simulink model "MATE_SynchronousMachineV2"  (R2024b)
settings: Solver=FixedStepDiscrete  StartTime=0.0  StopTime=6  FixedStep=Ts  RelTol=1e-4  EnableMultiTasking=on
PostLoadFcn:
  | Ts=25e-6;offset=4;
InitFcn:
  | Ts=25e-6;offset=4;
undefined symbols (not defined in the file): DiscIntNeverNeededParam, MATE, Phase, Rsnu, Single
libraries: fl_lib x76, nesl_utility x63, ee_lib x16, artemis x9, simetran x5, powerlib_extras x3, simulink_extras x2, simulink x2
(part 4 of 5)

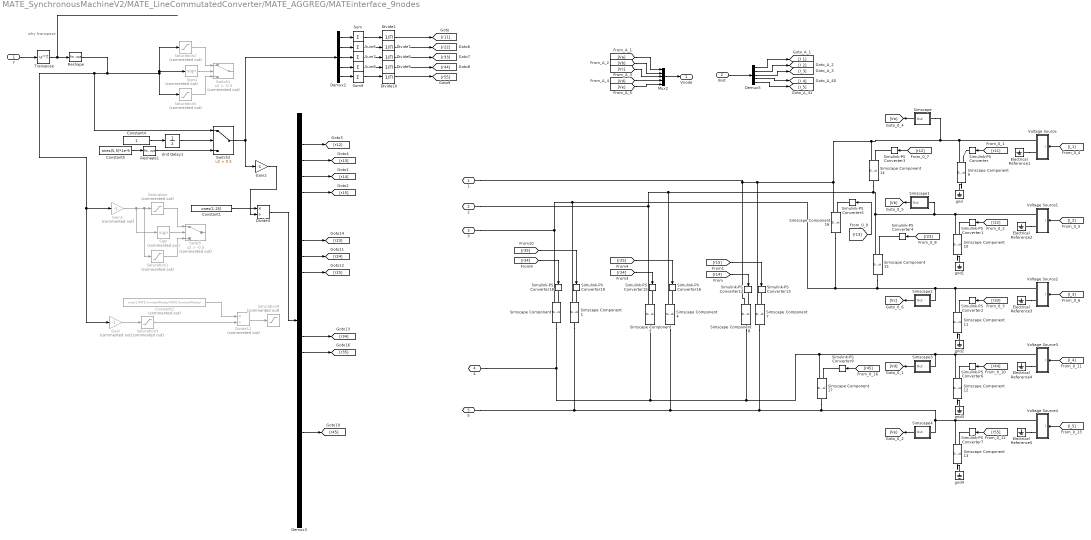
== system MATE_SynchronousMachineV2/MATE_LineCommutatedConverter/MATE_AGGREG/MATEinterface_9nodes ==
  note: why transpose
  Y : Inport
  Ihist : Inport  Port=2
  Constant1 : Constant  Value=ones(1,25)
  Constant2 : Constant  Commented=on  Value=ones(1,MATE.NumberOfNodes*MATE.NumberOfNodes)
  Constant4 : Constant
  Constant5 : Constant  Value=ones(5,5)*1e-9
  Demux2 : Demux  Outputs=[5 5 5 5 5]
      settings: DisplayOption=none
  Demux3 : Demux  Outputs=25
      settings: DisplayOption=none
  Demux5 : Demux  Outputs=[1 1 1 1 1]
      settings: DisplayOption=none
  Divide{1,7..10} (5 alike) : Product  Inputs=/
  Divide12 : Product  Commented=on  Inputs=*/  CollapseMode=Specified dimension
  Divide4 : Product  Inputs=*/  CollapseMode=Specified dimension
  Electrical Reference{1..5} (5 alike) : fl_lib/Electrical/Electrical Elements/Electrical Reference
  Gain : Gain  Commented=on  Gain=-1
  Gain1 : Gain  Commented=on  Gain=-1
  Gain2 : Gain  Gain=-1
  Mux2 : Mux  Inputs=[1 1 1 1 1]
  Reshape : Reshape
  Reshape1 : Reshape
  Saturation : Saturate  Commented=on  UpperLimit=1e12  LowerLimit=1e-12
  Saturation1 : Saturate  Commented=on  UpperLimit=-1e-12  LowerLimit=-1e12
  Saturation2 : Saturate  Commented=on  UpperLimit=1e12  LowerLimit=1e-12
  Saturation3 : Saturate  Commented=on  UpperLimit=1e15  LowerLimit=-1e15
  Saturation4 : Saturate  Commented=on  UpperLimit=1e15  LowerLimit=-1e15
  Saturation5 : Saturate  Commented=on  UpperLimit=-1e-12  LowerLimit=-1e12
  Sign : Signum  Commented=on
  Sign1 : Signum  Commented=on
  Simscape : Subsystem
      mask Display: disp('V')
  Simscape Component{,1,3..4,7..17} (15 alike) : SimscapeComponentBlock  SourceFile=variable_resistor_unlimited  ComponentPath=variable_resistor_unlimited  ComponentVariants="[\"variable_resistor_unlimited\"]"  ComponentVariantNames="[\"variable_resistor_unlimited\"]"  ClassName=variable_resistor_unlimited  SchemaVersion=1  R0=0 Ohm  Rmaxp=1e9 Ohm  Rmaxn=-1e9 Ohm  Rminp=1e-9 Ohm  Rminn=-1e-9 Ohm  i_specify=off  i_priority=None  i=0 A  i_nominal_specify=off  i_nominal_value=1  i_nominal_unit=A  v_specify=off  v_priority=None  v=0 V  v_nominal_specify=off  v_nominal_value=1  v_nominal_unit=V
      settings: CopyFcn=simscape.engine.sli.internal.componentblockcallback(gcbh,'COPY')  PreCopyFcn=simscape.engine.sli.internal.componentblockcallback(gcbh,'PRECOPY')  PreDeleteFcn=simscape.engine.sli.internal.componentblockcallback(gcbh,'PREDELETE')  InternalSimscapePortConfiguration="{\"Bottom\":[],\"Left\":[{\"id\":\"R\",\"label\":\"R\",\"type\":\"input\"},{\"id\":\"p\",\"label\":\"+\",\"type\":\"foundation.electrical.electrical\"}],\"Right\":[{\"id\":\"n\",\"label\":\"-\",\"type\":\"foundation.electrical.electrical\"}],\"Top\":[]}"
      mask Type: Variable Resistor
  Simscape1 : Subsystem
      mask Display: disp('V')
  Simscape2 : Subsystem
      mask Display: disp('V')
  Simscape3 : Subsystem
      mask Display: disp('V')
  Simscape4 : Subsystem
      mask Display: disp('V')
  Simulink-PS Converter{,1..7,9,12..13,15..16,18..19} (15 alike) : nesl_utility/Simulink-PS Converter  PhysicalDomain=network_engine_domain  SubClassName=ps_input  LeftPortType=input  RightPortType=output  PseudoPeriodic=off  Frequencies=[]  NoiseDistribution=none  NoiseParameters=[]  Unit=1  AffineConversion=off  FilteringAndDerivatives=provide  SimscapeFilterOrder=1  InputFilterTimeConstant=0.001  UdotUserProvided=0
  Sum{,6..9} (5 alike) : Sum  Inputs=+
  Switch : Switch  Commented=on  Criteria=u2 > Threshold  Threshold=-0.5  SaturateOnIntegerOverflow=off  InputSameDT=off
  Switch1 : Switch  Commented=on  Criteria=u2 > Threshold  Threshold=-0.5  SaturateOnIntegerOverflow=off  InputSameDT=off
  Switch2 : Switch  Criteria=u2 > Threshold  Threshold=0.5  SaturateOnIntegerOverflow=off  InputSameDT=off
  Transpose : Math  Operator=transpose
  Unit Delay1 : UnitDelay  SampleTime=Ts  HasFrameUpgradeWarning=on
  Voltage Source : Subsystem
  Voltage Source1 : Subsystem
  Voltage Source2 : Subsystem
  Voltage Source3 : Subsystem
  Voltage Source4 : Subsystem
  gnd{,1..4} (5 alike) : fl_lib/Electrical/Electrical Elements/Electrical Reference
  1 : PMIOPort  Side=Right
  2 : PMIOPort  Port=2  Side=Right
  3 : PMIOPort  Port=3  Side=Right
  4 : PMIOPort  Port=4  Side=Right
  5 : PMIOPort  Port=5  Side=Right
  Vnode : Outport  VectorParamsAs1DForOutWhenUnconnected=off
  wires:
  [I_2] -> Voltage Source1/1(I)
  Simscape2/1(Out) -> [Vc]
  [I_3] -> Voltage Source2/1(I)
  Simscape/1(Out) -> [Va]
  Simscape1/1(Out) -> [Vb]
  [I_1] -> Voltage Source/1(I)
  Y/1 -> Transpose/1
  Transpose/1 -> Reshape/1
  [r11] -> Simulink-PS Converter/1
  Sum/1 -> Divide1/1
  Divide1/1 -> [r11]
  [r22] -> Simulink-PS Converter1/1
  [r33] -> Simulink-PS Converter2/1
  [r12] -> Simulink-PS Converter3/1
  [r23] -> Simulink-PS Converter4/1
  [r13] -> Simulink-PS Converter5/1
  Demux2/1 -> Sum/1
  Divide7/1 -> [r22]
  Sum6/1 -> Divide7/1
  Demux2/2 -> Sum6/1
  Sum7/1 -> Divide8/1
  Divide8/1 -> [r33]
  Demux2/3 -> Sum7/1
  Demux2/4 -> Sum8/1
  Divide9/1 -> [r44]
  Sum8/1 -> Divide9/1
  Sum9/1 -> Divide10/1
  Divide10/1 -> [r55]
  Demux2/5 -> Sum9/1
  [r44] -> Simulink-PS Converter6/1
  [I_4] -> Voltage Source3/1(I)
  Simscape3/1(Out) -> [Vd]
  Simscape4/1(Out) -> [Ve]
  [I_5] -> Voltage Source4/1(I)
  [r55] -> Simulink-PS Converter7/1
  [r45] -> Simulink-PS Converter9/1
  [r14] -> Simulink-PS Converter12/1
  [r15] -> Simulink-PS Converter13/1
  [r25] -> Simulink-PS Converter16/1
  [r24] -> Simulink-PS Converter15/1
  Mux2/1 -> Vnode/1
  Ihist/1 -> Demux5/1
  Demux3/2 -> [r12]
  Demux3/3 -> [r13]
  Demux3/4 -> [r14]
  Demux3/5 -> [r15]
  Gain1/1 -> Sign/1, Saturation1/1, Saturation/1
  Constant1/1 -> Divide4/1
  [r35] -> Simulink-PS Converter19/1
  [r34] -> Simulink-PS Converter18/1
  Sign/1 -> Switch/2
  Saturation/1 -> Switch/1
  Saturation1/1 -> Switch/3
  Divide12/1 -> Saturation4/1
  Saturation3/1 -> Divide12/2
  Constant2/1 -> Divide12/1
  Gain/1 -> Saturation3/1
  Saturation5/1 -> Switch1/3
  Saturation2/1 -> Switch1/1
  Sign1/1 -> Switch1/2
  Reshape/1 -> Gain1/1, Gain/1, Switch2/1, Saturation2/1, Sign1/1, Saturation5/1
  Unit Delay1/1 -> Switch2/2
  Constant4/1 -> Unit Delay1/1
  Reshape1/1 -> Switch2/3
  Gain2/1 -> Divide4/2
  Demux5/4 -> [I_4]
  Demux5/3 -> [I_3]
  Demux5/5 -> [I_5]
  Demux5/2 -> [I_2]
  Demux5/1 -> [I_1]
  [Vd] -> Mux2/4
  [Ve] -> Mux2/5
  [Vc] -> Mux2/3
  [Vb] -> Mux2/2
  [Va] -> Mux2/1
  Demux3/8 -> [r23]
  Demux3/9 -> [r24]
  Demux3/10 -> [r25]
  Demux3/14 -> [r34]
  Demux3/15 -> [r35]
  Demux3/20 -> [r45]
  Constant5/1 -> Reshape1/1
  Switch2/1 -> Demux2/1, Gain2/1
  Divide4/1 -> Demux3/1
  connections:
  Simscape Component14/LConn2 -- Simscape Component9/LConn2 -- Voltage Source/RConn1 -- Simscape/LConn1 -- Simscape Component16/LConn2 -- Simscape Component7/LConn2 -- 1/RConn1 -- Simscape Component8/LConn2
  Simscape Component11/LConn2 -- Voltage Source2/RConn1 -- Simscape2/LConn1 -- Simscape Component15/RConn1 -- Simscape Component16/RConn1 -- Simscape Component1/LConn2 -- Simscape Component/LConn2 -- 3/RConn1
  Simscape Component10/LConn2 -- Voltage Source1/RConn1 -- Simscape1/LConn1 -- Simscape Component15/LConn2 -- Simscape Component14/RConn1 -- Simscape Component4/LConn2 -- Simscape Component3/LConn2 -- 2/RConn1
  Electrical Reference2/LConn1 -- Voltage Source1/RConn2
  Electrical Reference3/LConn1 -- Voltage Source2/RConn2
  Electrical Reference1/LConn1 -- Voltage Source/RConn2
  Simscape Component9/RConn1 -- gnd/LConn1
  Simscape Component9/LConn1 -- Simulink-PS Converter/RConn1
  Simscape Component10/RConn1 -- gnd1/LConn1
  Simscape Component10/LConn1 -- Simulink-PS Converter1/RConn1
  Simscape Component11/RConn1 -- gnd2/LConn1
  Simscape Component11/LConn1 -- Simulink-PS Converter2/RConn1
  Simscape Component14/LConn1 -- Simulink-PS Converter3/RConn1
  Simscape Component15/LConn1 -- Simulink-PS Converter4/RConn1
  Simscape Component16/LConn1 -- Simulink-PS Converter5/RConn1
  Simscape Component17/LConn2 -- 4/RConn1 -- Simscape Component/RConn1 -- Simscape Component3/RConn1 -- Simscape Component8/RConn1 -- Simscape Component12/LConn2 -- Voltage Source3/RConn1 -- Simscape3/LConn1
  Simscape Component12/LConn1 -- Simulink-PS Converter6/RConn1
  Simscape Component12/RConn1 -- gnd3/LConn1
  Electrical Reference4/LConn1 -- Voltage Source3/RConn2
  Simscape Component13/LConn2 -- Voltage Source4/RConn1 -- Simscape Component17/RConn1 -- Simscape Component1/RConn1 -- 5/RConn1 -- Simscape Component4/RConn1 -- Simscape Component7/RConn1 -- Simscape4/LConn1
  Simscape Component13/RConn1 -- gnd4/LConn1
  Simscape Component13/LConn1 -- Simulink-PS Converter7/RConn1
  Electrical Reference5/LConn1 -- Voltage Source4/RConn2
  Simscape Component17/LConn1 -- Simulink-PS Converter9/RConn1
  Simscape Component8/LConn1 -- Simulink-PS Converter12/RConn1
  Simscape Component7/LConn1 -- Simulink-PS Converter13/RConn1
  Simscape Component3/LConn1 -- Simulink-PS Converter15/RConn1
  Simscape Component4/LConn1 -- Simulink-PS Converter16/RConn1
  Simscape Component/LConn1 -- Simulink-PS Converter18/RConn1
  Simscape Component1/LConn1 -- Simulink-PS Converter19/RConn1

== system MATE_SynchronousMachineV2/MATE_LineCommutatedConverter/MATE_AGGREG/Subsystem ==
  note: yout=[ 'U_XX/Th1 ' 'U_XX/Th2 ' 'U_XX/Th3 ' 'U_XX/Th4 ' 'U_XX/Th5 ' 'U_XX/Th6 ' 'U_MATE+/vm' 'U_MATE-/vm' 'U_MATEA/vm' 'U_MATEB/vm' 'U_MATEC/vm'];
  A : PMIOPort  Side=Left
  -1 : PMIOPort  Port=2  Side=Right
  B : PMIOPort  Port=3  Side=Left
  -2 : PMIOPort  Port=4  Side=Right
  C : PMIOPort  Port=5  Side=Left
  -3 : PMIOPort  Port=6  Side=Right
  + : PMIOPort  Port=7  Side=Left
  -4 : PMIOPort  Port=8  Side=Right
  - : PMIOPort  Port=9  Side=Left
  -5 : PMIOPort  Port=10  Side=Right
  connections:
  +/RConn1 -- -1/RConn1
  -/RConn1 -- -2/RConn1
  A/RConn1 -- -3/RConn1
  B/RConn1 -- -4/RConn1
  C/RConn1 -- -5/RConn1

== system MATE_SynchronousMachineV2/turbine1/Hydraulic Turbine and Governor/Model ==
  wref : Inport
  Pref : Inport  Port=2
  we : Inport  Port=3
  Pe : Inport  Port=4
  dw : Inport  Port=5
  Constant1 : Constant  Value=dref
  Discrete PID Controller : Subsystem  mask(Discrete PID Controller){Kp=kp, Ki=ki, Kd=kd, TcD=td, Par_Limits=[1e6 -1e6], Init=go, Ts=Ts}
      mask prompts: Kp "Proportional gain (Kp):"; Ki "Integral gain (Ki):"; Kd "Derivative gain (Kd):"; TcD "Time constant for derivative (s):"; Par_Limits "Output limits: [ Upper   Lower ]"; Init "Output initial value:"; Ts "Sample time:"
      mask help: This block implements a discrete PID controller.
      mask init:
      | UpperLimit=Par_Limits(1);
      | LowerLimit=Par_Limits(2);
      mask Display: disp('PID');
  Sum : Sum  Inputs=+-  InputSameDT=on  SaturateOnIntegerOverflow=on  OutDataTypeStr=Inherit: Same as first input
  Sum1 : Sum  Inputs=+-  InputSameDT=on  SaturateOnIntegerOverflow=on  OutDataTypeStr=Inherit: Same as first input
  Sum5 : Sum  Inputs=-+  InputSameDT=on  SaturateOnIntegerOverflow=on  OutDataTypeStr=Inherit: Same as first input
  Switch : Switch  Threshold=0.5  SaturateOnIntegerOverflow=off
  permanent droop : Gain  Gain=Rp  SaturateOnIntegerOverflow=on  OutDataTypeStr=Inherit: Same as input  ParamDataTypeStr=Inherit: Same as input
  servo-motor : Subsystem
      mask Display: disp('servo-\nmotor')
  turbine : Subsystem
      mask Display: disp('hydraulic\nturbine')
  Pm : Outport  InitialOutput=0
  gate : Outport  Port=2  InitialOutput=0
  wires:
  Constant1/1 -> Switch/2
  Switch/1 -> permanent droop/1
  Pe/1 -> Sum5/2
  Pref/1 -> Sum5/1
  Sum1/1 -> Discrete PID Controller/1(Error)
  permanent droop/1 -> Sum1/2
  Sum/1 -> Sum1/1
  Discrete PID Controller/1(Out) -> servo-motor/1(regulator's output)
  wref/1 -> Sum/1
  we/1 -> Sum/2
  Sum5/1 -> Switch/3
  servo-motor/1(gate opening) -> turbine/2(gate opening), gate/1, Switch/1
  dw/1 -> turbine/1(dw)
  turbine/1(Pm) -> Pm/1

== system MATE_SynchronousMachineV2/turbine1/Mechanical model/Delay Prediction ==
  in : Inport
  F2 : Gain  Gain=2  SaturateOnIntegerOverflow=on  OutDataTypeStr=Inherit: Same as input  ParamDataTypeStr=Inherit: Same as input
  Sum1 : Sum  Inputs=+-  InputSameDT=on  SaturateOnIntegerOverflow=on  OutDataTypeStr=Inherit: Same as first input
  dw_delay : UnitDelay  SampleTime=Ts  HasFrameUpgradeWarning=on
  dw_predict : UnitDelay  SampleTime=Ts  HasFrameUpgradeWarning=on
  dw : Outport
  wires:
  dw_delay/1 -> dw_predict/1, F2/1
  in/1 -> dw_delay/1
  dw_predict/1 -> Sum1/2
  F2/1 -> Sum1/1
  Sum1/1 -> dw/1

== system MATE_SynchronousMachineV2/Command/Regulateur de tension (Mode automatique)/Discrete 3-phase Positive-Sequence Fundamental Value/Discrete Mean value1 ==
  note: Discrete Mean Value
  In : Inport
  Constant : Constant  Value=Vinit  SampleTime=Ts
  Discrete Variable Transport Delay : powerlib_extras/Discrete  Control Blocks/Discrete Variable Transport Delay  MaxDelay=Delay+Ts  InitialValue=0  Ts=Ts
  Gain : Gain  Gain=K1  SaturateOnIntegerOverflow=on  OutDataTypeStr=Inherit: Same as input  ParamDataTypeStr=Inherit: Same as input
  Gain1 : Gain  Gain=K2  SaturateOnIntegerOverflow=on  OutDataTypeStr=Inherit: Same as input  ParamDataTypeStr=Inherit: Same as input
  Integ4 : DiscreteIntegrator  IntegratorMethod=Integration: Trapezoidal  SampleTime=Ts  ICPrevOutput=DiscIntNeverNeededParam  ICPrevScaledInput=DiscIntNeverNeededParam
  K1 : Constant  Value=Delay  SampleTime=Ts
  K2 : Constant  Value=Freq  SampleTime=Ts
  Product : Product  InputSameDT=on  SaturateOnIntegerOverflow=on  OutDataTypeStr=Inherit: Same as first input
  Step : Step  Time=1/Freq  SampleTime=Ts
  Sum1 : Sum  Inputs=+-  InputSameDT=on  SaturateOnIntegerOverflow=on  OutDataTypeStr=Inherit: Same as first input
  Sum5 : Sum  InputSameDT=on  SaturateOnIntegerOverflow=on  OutDataTypeStr=Inherit: Same as first input
  Sum7 : Sum  Inputs=-+  InputSameDT=on  SaturateOnIntegerOverflow=on  OutDataTypeStr=Inherit: Same as first input
  Switch : Switch  Threshold=0.5  SaturateOnIntegerOverflow=off
  Unit Delay : UnitDelay  SampleTime=Ts  HasFrameUpgradeWarning=on
  Mean : Outport  VectorParamsAs1DForOutWhenUnconnected=off
  wires:
  Product/1 -> Sum5/1  "Mean value"
  Sum7/1 -> Product/1
  Integ4/1 -> Discrete Variable Transport Delay/1, Sum7/2
  K2/1 -> Product/2
  In/1 -> Integ4/1, Gain1/1, Unit Delay/1  "In"
  Sum5/1 -> Switch/1
  Step/1 -> Switch/2
  Constant/1 -> Switch/3
  Switch/1 -> Mean/1
  Discrete Variable Transport Delay/1 -> Sum7/1
  K1/1 -> Discrete Variable Transport Delay/2
  Gain1/1 -> Sum1/1
  Unit Delay/1 -> Gain/1
  Gain/1 -> Sum1/2
  Sum1/1 -> Sum5/2  "Correction"

== system MATE_SynchronousMachineV2/Command/Regulateur de tension (Mode automatique)/Discrete 3-phase Positive-Sequence Fundamental Value/Discrete Mean value3 ==
  note: Discrete Mean Value
  In : Inport
  Constant : Constant  Value=Vinit  SampleTime=Ts
  Discrete Variable Transport Delay : powerlib_extras/Discrete  Control Blocks/Discrete Variable Transport Delay  MaxDelay=Delay+Ts  InitialValue=0  Ts=Ts
  Gain : Gain  Gain=K1  SaturateOnIntegerOverflow=on  OutDataTypeStr=Inherit: Same as input  ParamDataTypeStr=Inherit: Same as input
  Gain1 : Gain  Gain=K2  SaturateOnIntegerOverflow=on  OutDataTypeStr=Inherit: Same as input  ParamDataTypeStr=Inherit: Same as input
  Integ4 : DiscreteIntegrator  IntegratorMethod=Integration: Trapezoidal  SampleTime=Ts  ICPrevOutput=DiscIntNeverNeededParam  ICPrevScaledInput=DiscIntNeverNeededParam
  K1 : Constant  Value=Delay  SampleTime=Ts
  K2 : Constant  Value=Freq  SampleTime=Ts
  Product : Product  InputSameDT=on  SaturateOnIntegerOverflow=on  OutDataTypeStr=Inherit: Same as first input
  Step : Step  Time=1/Freq  SampleTime=Ts
  Sum1 : Sum  Inputs=+-  InputSameDT=on  SaturateOnIntegerOverflow=on  OutDataTypeStr=Inherit: Same as first input
  Sum5 : Sum  InputSameDT=on  SaturateOnIntegerOverflow=on  OutDataTypeStr=Inherit: Same as first input
  Sum7 : Sum  Inputs=-+  InputSameDT=on  SaturateOnIntegerOverflow=on  OutDataTypeStr=Inherit: Same as first input
  Switch : Switch  Threshold=0.5  SaturateOnIntegerOverflow=off
  Unit Delay : UnitDelay  SampleTime=Ts  HasFrameUpgradeWarning=on
  Mean : Outport  VectorParamsAs1DForOutWhenUnconnected=off
  wires:
  Sum1/1 -> Sum5/2  "Correction"
  Gain/1 -> Sum1/2
  Unit Delay/1 -> Gain/1
  Gain1/1 -> Sum1/1
  K1/1 -> Discrete Variable Transport Delay/2
  Discrete Variable Transport Delay/1 -> Sum7/1
  Switch/1 -> Mean/1
  Constant/1 -> Switch/3
  Step/1 -> Switch/2
  Sum5/1 -> Switch/1
  In/1 -> Unit Delay/1, Gain1/1, Integ4/1  "In"
  K2/1 -> Product/2
  Integ4/1 -> Sum7/2, Discrete Variable Transport Delay/1
  Sum7/1 -> Product/1
  Product/1 -> Sum5/1  "Mean value"

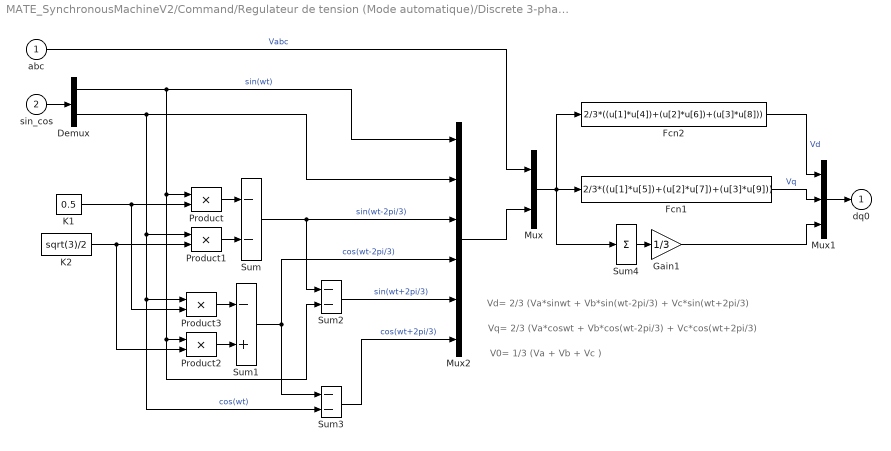
== system MATE_SynchronousMachineV2/Command/Regulateur de tension (Mode automatique)/Discrete 3-phase Positive-Sequence Fundamental Value/abc_to_dq0 Transformation ==
  note: V0= 1/3 (Va + Vb + Vc )
  note: Vd= 2/3 (Va*sinwt + Vb*sin(wt-2pi/3) + Vc*sin(wt+2pi/3)
  note: Vq= 2/3 (Va*coswt + Vb*cos(wt-2pi/3) + Vc*cos(wt+2pi/3)
  abc : Inport  PortDimensions=3
  sin_cos : Inport  Port=2  PortDimensions=2
  Demux : Demux  Outputs=2
  Fcn1 : Fcn  Expr=2/3*((u[1]*u[5])+(u[2]*u[7])+(u[3]*u[9]))
  Fcn2 : Fcn  Expr=2/3*((u[1]*u[4])+(u[2]*u[6])+(u[3]*u[8]))
  Gain1 : Gain  Gain=1/3  SaturateOnIntegerOverflow=on  OutDataTypeStr=Inherit: Same as input  ParamDataTypeStr=Inherit: Same as input
  K1 : Constant  Value=0.5
  K2 : Constant  Value=sqrt(3)/2
  Mux : Mux  Inputs=2
  Mux1 : Mux  Inputs=3
  Mux2 : Mux  Inputs=6
  Product{,1..3} (4 alike) : Product  InputSameDT=on  SaturateOnIntegerOverflow=on  OutDataTypeStr=Inherit: Same as first input
  Sum : Sum  Inputs=--  InputSameDT=on  SaturateOnIntegerOverflow=on  OutDataTypeStr=Inherit: Same as first input
  Sum1 : Sum  Inputs=-+  InputSameDT=on  SaturateOnIntegerOverflow=on  OutDataTypeStr=Inherit: Same as first input
  Sum2 : Sum  Inputs=--  InputSameDT=on  SaturateOnIntegerOverflow=on  OutDataTypeStr=Inherit: Same as first input
  Sum3 : Sum  Inputs=--  InputSameDT=on  SaturateOnIntegerOverflow=on  OutDataTypeStr=Inherit: Same as first input
  Sum4 : Sum  Inputs=1  InputSameDT=on  SaturateOnIntegerOverflow=on  OutDataTypeStr=Inherit: Same as first input
  dq0 : Outport  InitialOutput=0  VectorParamsAs1DForOutWhenUnconnected=off
  wires:
  Gain1/1 -> Mux1/3
  Fcn2/1 -> Mux1/1  "Vd"
  Fcn1/1 -> Mux1/2  "Vq"
  Mux1/1 -> dq0/1
  Sum4/1 -> Gain1/1
  Mux/1 -> Sum4/1, Fcn1/1, Fcn2/1
  Sum1/1 -> Sum3/1, Mux2/4  "cos(wt-2pi/3)"
  Sum/1 -> Sum2/1, Mux2/3  "sin(wt-2pi/3)"
  K2/1 -> Product2/2, Product1/2
  K1/1 -> Product3/2, Product/2
  Sum2/1 -> Mux2/5  "sin(wt+2pi/3)"
  Sum3/1 -> Mux2/6  "cos(wt+2pi/3)"
  Product2/1 -> Sum1/2
  Product3/1 -> Sum1/1
  Product1/1 -> Sum/2
  Product/1 -> Sum/1
  Demux/1 -> Mux2/1, Sum2/2, Product2/1, Product/1  "sin(wt)"
  Demux/2 -> Mux2/2, Product1/1, Product3/1, Sum3/2  "cos(wt)"
  sin_cos/1 -> Demux/1
  Mux2/1 -> Mux/2
  abc/1 -> Mux/1  "Vabc"

== system MATE_SynchronousMachineV2/Command/Synchro Generateur d'mpulsions /Discrete 3-phase PLL/2nd-Order Filter ==
  In : Inport
  Discrete State-Space : DiscreteStateSpace  A=Ad  B=Bd  C=Cd  D=Dd  InitialCondition=x0d  SampleTime=Ts
  Out : Outport  InitialOutput=0  VectorParamsAs1DForOutWhenUnconnected=off
  wires:
  Discrete State-Space/1 -> Out/1
  In/1 -> Discrete State-Space/1

== system MATE_SynchronousMachineV2/Command/Synchro Generateur d'mpulsions /Discrete 3-phase PLL/Automatic Gain Control ==
  Freq : Inport
  Sin_Cos : Inport  Port=2
  Vabc : Inport  Port=3
  Enable : EnablePort  PropagateVarSize=During execution
  3-phase PLL-Driven Positive-Sequence Fundamental Value : Subsystem  mask(Discrete 3-phase PLL-Driven Positive-Sequence Fundamental Value){Finit=Finit, Fmin=Fmin, Par_Init=[1 0], Ts=Ts}
      mask prompts: Finit "Initial frequency (Hz):"; Fmin "Minimum frequency (Hz):"; Par_Init "Initial input (positive component): [ Mag  Phase-relative-to-PLL(degrees) ]"; Ts "Sample time:"
      mask help:
      | Compute the positive-sequence component of the input 3 signal over a running window of one cycle of fundamental frequency given by input 1. The signal can be a set of three balanced or unbalanced signals which may contain harmonics.
      | The reference frame required for the computation is given by the input 2 (a two-dimension signal).
      |
      | The two outputs return respectively the magnitude (same units as the input 3 signal) and phase (in degrees relative to the PLL phase) of the fundamental.
      |
      | For the first cycle of simulation, the outputs are held constant to the values specified by the Initial input parameter. The Minimum frequency parameter is used to determine the buffer size of the Variable Transport Delay block used in the model.
      mask init:
      | Real_Init=Par_Init(1)*cos(pi/180*Par_Init(2));
      | Imag_Init=Par_Init(1)*sin(pi/180*Par_Init(2));
      mask Display: disp('')
  Math Function : Math  Operator=reciprocal  SignedPower=on
  Saturation : Saturate  UpperLimit=2  LowerLimit=0.01
  Terminator : Terminator
  Gain : Outport  InitialOutput=[1]  VectorParamsAs1DForOutWhenUnconnected=off
  wires:
  3-phase PLL-Driven Positive-Sequence Fundamental Value/2(Phase) -> Terminator/1
  Saturation/1 -> Math Function/1
  3-phase PLL-Driven Positive-Sequence Fundamental Value/1(Mag) -> Saturation/1
  Freq/1 -> 3-phase PLL-Driven Positive-Sequence Fundamental Value/1(Freq)
  Sin_Cos/1 -> 3-phase PLL-Driven Positive-Sequence Fundamental Value/2(Sin_Cos)
  Vabc/1 -> 3-phase PLL-Driven Positive-Sequence Fundamental Value/3(abc)
  Math Function/1 -> Gain/1

== system MATE_SynchronousMachineV2/Command/Synchro Generateur d'mpulsions /Discrete 3-phase PLL/Controller ==
  Error : Inport
  Discrete Derivative : simulink/Discrete/Discrete Derivative  gainval=1.0  ICPrevScaledInput=0.0  OutMin=[]  OutMax=[]  OutDataType=sfix(16)  OutScaling=2^-10  DoSatur=off
  Discrete-Time Integrator : DiscreteIntegrator  InitialCondition=Init  SampleTime=Ts  LimitOutput=on  UpperSaturationLimit=UpperLimit  LowerSaturationLimit=LowerLimit  ICPrevOutput=DiscIntNeverNeededParam  ICPrevScaledInput=DiscIntNeverNeededParam
  Kp4 : Gain  Gain=Kp  SaturateOnIntegerOverflow=on  OutDataTypeStr=Inherit: Same as input  ParamDataTypeStr=Inherit: Same as input
  Kp5 : Gain  Gain=Ki  SaturateOnIntegerOverflow=on  OutDataTypeStr=Inherit: Same as input  ParamDataTypeStr=Inherit: Same as input
  Kp6 : Gain  Gain=Kd  SaturateOnIntegerOverflow=on  OutDataTypeStr=Inherit: Same as input  ParamDataTypeStr=Inherit: Same as input
  Saturation2 : Saturate  UpperLimit=UpperLimit  LowerLimit=LowerLimit
  Sum6 : Sum  Inputs=+++  InputSameDT=on  SaturateOnIntegerOverflow=on  OutDataTypeStr=Inherit: Same as first input
  Zero-Order Hold : ZeroOrderHold  SampleTime=Ts
  Out : Outport  InitialOutput=0  VectorParamsAs1DForOutWhenUnconnected=off
  wires:
  Error/1 -> Kp4/1, Kp5/1, Kp6/1
  Sum6/1 -> Saturation2/1
  Kp5/1 -> Discrete-Time Integrator/1
  Kp6/1 -> Zero-Order Hold/1
  Kp4/1 -> Sum6/1
  Discrete-Time Integrator/1 -> Sum6/2
  Discrete Derivative/1 -> Sum6/3
  Saturation2/1 -> Out/1
  Zero-Order Hold/1 -> Discrete Derivative/1

== system MATE_SynchronousMachineV2/Command/Synchro Generateur d'mpulsions /Discrete 3-phase PLL/Discrete Rate Limiter ==
  note: Beat Ronner
      | ABB Industrie AG
      | Turgi, Switzerland
  note: Delta(u)
  In : Inport
  Saturation : Saturate  UpperLimit=UpperLimit  LowerLimit=LowerLimit
  Sum : Sum  Inputs=|++  InputSameDT=on  SaturateOnIntegerOverflow=on  OutDataTypeStr=Inherit: Same as first input
  Sum1 : Sum  Inputs=|+-  InputSameDT=on  SaturateOnIntegerOverflow=on  OutDataTypeStr=Inherit: Same as first input
  Unit Delay : UnitDelay  InitialCondition=Vinit  SampleTime=Ts  HasFrameUpgradeWarning=on
  Out : Outport  VectorParamsAs1DForOutWhenUnconnected=off
  wires:
  Unit Delay/1 -> Sum/2, Sum1/2  "y-1"
  Sum/1 -> Unit Delay/1, Out/1  "y"
  Saturation/1 -> Sum/1  "Delta(u)_limit"
  Sum1/1 -> Saturation/1
  In/1 -> Sum1/1  "u"

== system MATE_SynchronousMachineV2/Command/Synchro Generateur d'mpulsions /Discrete 3-phase PLL/Variable Frequency Mean value ==
  Freq : Inport  PortDimensions=1
  In : Inport  Port=2  PortDimensions=1
  Constant : Constant  Value=Vinit  SampleTime=Ts
  Correction subsystem : Subsystem
  Discrete Variable Transport Delay : Subsystem  mask(Discrete variable transport delay){MaxDelay=MaxDelay, InitialValue=0, Ts=Ts}
      mask prompts: MaxDelay "Maximum delay (s):"; InitialValue "Initial input:"; Ts "Sample time:"
      mask help:
      | Apply a delay to the first input (In) signal.
      | The second input (D) specifies the delay time.
  Gain : Gain  Gain=Ts  SaturateOnIntegerOverflow=on  OutDataTypeStr=Inherit: Same as input  ParamDataTypeStr=Inherit: Same as input
  Integ4 : DiscreteIntegrator  IntegratorMethod=Integration: Trapezoidal  SampleTime=Ts  ICPrevOutput=DiscIntNeverNeededParam  ICPrevScaledInput=DiscIntNeverNeededParam
  Number of samples per cycle : Fcn  Expr=1/u[1]/Ts
  Product : Product  InputSameDT=on  SaturateOnIntegerOverflow=on  OutDataTypeStr=Inherit: Same as first input
  Rounding Function : Rounding  Operator=ceil
  Step : Step  Time=1/Finit  SampleTime=Ts
  Sum5 : Sum  InputSameDT=on  SaturateOnIntegerOverflow=on  OutDataTypeStr=Inherit: Same as first input
  Sum7 : Sum  Inputs=-+  InputSameDT=on  SaturateOnIntegerOverflow=on  OutDataTypeStr=Inherit: Same as first input
  Switch : Switch  Threshold=0.5  SaturateOnIntegerOverflow=off
  To avoid division by zero : Saturate  UpperLimit=1e6  LowerLimit=1e-6
  Mean : Outport  VectorParamsAs1DForOutWhenUnconnected=off
  wires:
  In/1 -> Integ4/1, Correction subsystem/3(In)  "In"
  Product/1 -> Sum5/1  "Mean value"
  Discrete Variable Transport Delay/1(Out) -> Sum7/1
  Sum7/1 -> Product/1
  Integ4/1 -> Discrete Variable Transport Delay/1(In), Sum7/2
  Freq/1 -> Product/2, To avoid division by zero/1  "Freq"
  Gain/1 -> Discrete Variable Transport Delay/2(D)  "Delay"
  Rounding Function/1 -> Gain/1, Correction subsystem/2(F)
  Number of samples per cycle/1 -> Rounding Function/1, Correction subsystem/1(N)
  Sum5/1 -> Switch/1
  Constant/1 -> Switch/3
  Switch/1 -> Mean/1
  To avoid division by zero/1 -> Number of samples per cycle/1  "Freq"
  Correction subsystem/1(Out) -> Sum5/2
  Step/1 -> Switch/2

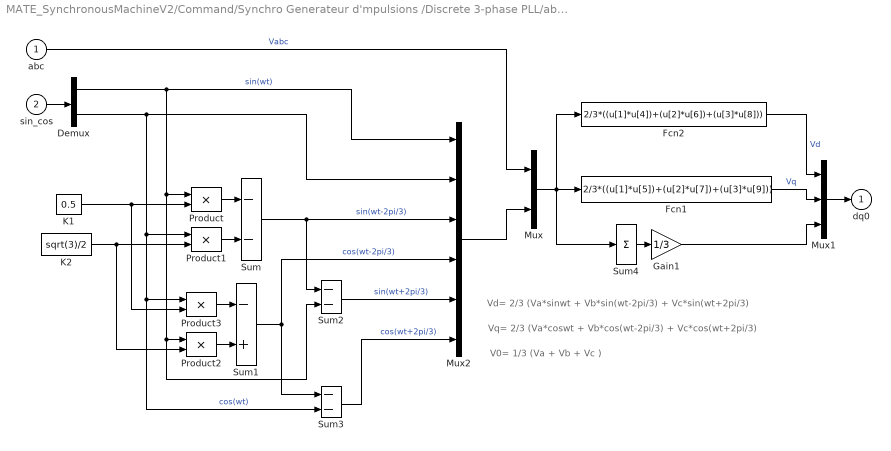
== system MATE_SynchronousMachineV2/Command/Synchro Generateur d'mpulsions /Discrete 3-phase PLL/abc_to_dq0 Transformation ==
  note: V0= 1/3 (Va + Vb + Vc )
  note: Vd= 2/3 (Va*sinwt + Vb*sin(wt-2pi/3) + Vc*sin(wt+2pi/3)
  note: Vq= 2/3 (Va*coswt + Vb*cos(wt-2pi/3) + Vc*cos(wt+2pi/3)
  abc : Inport  PortDimensions=3
  sin_cos : Inport  Port=2  PortDimensions=2
  Demux : Demux  Outputs=2
  Fcn1 : Fcn  Expr=2/3*((u[1]*u[5])+(u[2]*u[7])+(u[3]*u[9]))
  Fcn2 : Fcn  Expr=2/3*((u[1]*u[4])+(u[2]*u[6])+(u[3]*u[8]))
  Gain1 : Gain  Gain=1/3  SaturateOnIntegerOverflow=on  OutDataTypeStr=Inherit: Same as input  ParamDataTypeStr=Inherit: Same as input
  K1 : Constant  Value=0.5
  K2 : Constant  Value=sqrt(3)/2
  Mux : Mux  Inputs=2
  Mux1 : Mux  Inputs=3
  Mux2 : Mux  Inputs=6
  Product{,1..3} (4 alike) : Product  InputSameDT=on  SaturateOnIntegerOverflow=on  OutDataTypeStr=Inherit: Same as first input
  Sum : Sum  Inputs=--  InputSameDT=on  SaturateOnIntegerOverflow=on  OutDataTypeStr=Inherit: Same as first input
  Sum1 : Sum  Inputs=-+  InputSameDT=on  SaturateOnIntegerOverflow=on  OutDataTypeStr=Inherit: Same as first input
  Sum2 : Sum  Inputs=--  InputSameDT=on  SaturateOnIntegerOverflow=on  OutDataTypeStr=Inherit: Same as first input
  Sum3 : Sum  Inputs=--  InputSameDT=on  SaturateOnIntegerOverflow=on  OutDataTypeStr=Inherit: Same as first input
  Sum4 : Sum  Inputs=1  InputSameDT=on  SaturateOnIntegerOverflow=on  OutDataTypeStr=Inherit: Same as first input
  dq0 : Outport  InitialOutput=0  VectorParamsAs1DForOutWhenUnconnected=off
  wires:
  Gain1/1 -> Mux1/3
  Fcn2/1 -> Mux1/1  "Vd"
  Fcn1/1 -> Mux1/2  "Vq"
  Mux1/1 -> dq0/1
  Sum4/1 -> Gain1/1
  Mux/1 -> Sum4/1, Fcn1/1, Fcn2/1
  Sum1/1 -> Sum3/1, Mux2/4  "cos(wt-2pi/3)"
  Sum/1 -> Sum2/1, Mux2/3  "sin(wt-2pi/3)"
  K2/1 -> Product2/2, Product1/2
  K1/1 -> Product3/2, Product/2
  Sum2/1 -> Mux2/5  "sin(wt+2pi/3)"
  Sum3/1 -> Mux2/6  "cos(wt+2pi/3)"
  Product2/1 -> Sum1/2
  Product3/1 -> Sum1/1
  Product1/1 -> Sum/2
  Product/1 -> Sum/1
  Demux/1 -> Mux2/1, Sum2/2, Product2/1, Product/1  "sin(wt)"
  Demux/2 -> Mux2/2, Product1/1, Product3/1, Sum3/2  "cos(wt)"
  sin_cos/1 -> Demux/1
  Mux2/1 -> Mux/2
  abc/1 -> Mux/1  "Vabc"

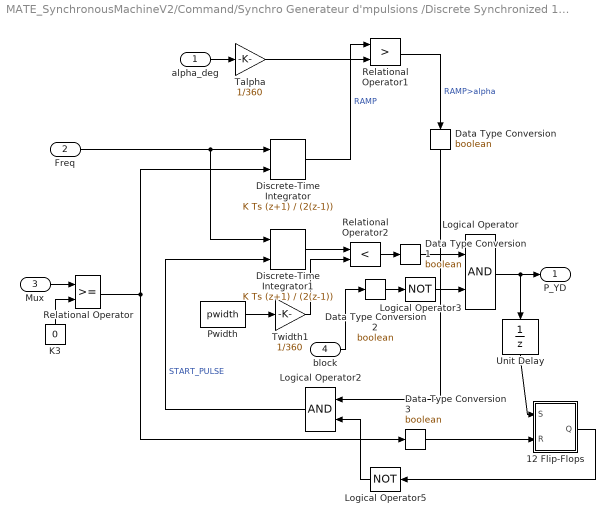
== system MATE_SynchronousMachineV2/Command/Synchro Generateur d'mpulsions /Discrete Synchronized 12-Pulse Generator/Pulse generation ==
  alpha_deg : Inport
  Freq : Inport  Port=2
  Mux : Inport  Port=3
  block : Inport  Port=4
  12 Flip-Flops : Subsystem
  Data Type Conversion{,1..3} (4 alike) : DataTypeConversion  OutDataTypeStr=boolean
  Discrete-Time Integrator : DiscreteIntegrator  IntegratorMethod=Integration: Trapezoidal  ExternalReset=rising  SampleTime=Ts  ICPrevOutput=DiscIntNeverNeededParam  ICPrevScaledInput=DiscIntNeverNeededParam
  Discrete-Time Integrator1 : DiscreteIntegrator  IntegratorMethod=Integration: Trapezoidal  ExternalReset=rising  SampleTime=Ts  ICPrevOutput=DiscIntNeverNeededParam  ICPrevScaledInput=DiscIntNeverNeededParam
  K3 : Constant  Value=0
  Logical Operator : Logic
  Logical Operator2 : Logic
  Logical Operator3 : Logic  Operator=NOT  Inputs=1
  Logical Operator5 : Logic  Operator=NOT  Inputs=1
  Pwidth : Constant  Value=pwidth
  Relational Operator : RelationalOperator
  Relational Operator1 : RelationalOperator  Operator=>
  Relational Operator2 : RelationalOperator  Operator=<
  Talpha : Gain  Gain=1/360  SaturateOnIntegerOverflow=on  OutDataTypeStr=Inherit: Same as input  ParamDataTypeStr=Inherit: Same as input
  Twidth1 : Gain  Gain=1/360  SaturateOnIntegerOverflow=on  OutDataTypeStr=Inherit: Same as input  ParamDataTypeStr=Inherit: Same as input
  Unit Delay : UnitDelay  SampleTime=Ts  HasFrameUpgradeWarning=on
  P_YD : Outport  VectorParamsAs1DForOutWhenUnconnected=off
  wires:
  block/1 -> Data Type Conversion2/1
  Mux/1 -> Relational Operator/1
  alpha_deg/1 -> Talpha/1
  Freq/1 -> Discrete-Time Integrator1/1, Discrete-Time Integrator/1
  K3/1 -> Relational Operator/2
  Discrete-Time Integrator/1 -> Relational Operator1/1  "RAMP"
  Talpha/1 -> Relational Operator1/2
  Discrete-Time Integrator1/1 -> Relational Operator2/1
  Twidth1/1 -> Relational Operator2/2
  Logical Operator2/1 -> Discrete-Time Integrator1/2  "START_PULSE"
  Logical Operator5/1 -> Logical Operator2/2
  Relational Operator/1 -> Discrete-Time Integrator/2, Data Type Conversion3/1
  Pwidth/1 -> Twidth1/1
  Logical Operator3/1 -> Logical Operator/2
  12 Flip-Flops/1(Q) -> Logical Operator5/1
  Logical Operator/1 -> P_YD/1, Unit Delay/1
  Unit Delay/1 -> 12 Flip-Flops/1(S)
  Relational Operator1/1 -> Data Type Conversion/1  "RAMP>alpha"
  Data Type Conversion/1 -> Logical Operator2/1
  Relational Operator2/1 -> Data Type Conversion1/1
  Data Type Conversion1/1 -> Logical Operator/1
  Data Type Conversion2/1 -> Logical Operator3/1
  Data Type Conversion3/1 -> 12 Flip-Flops/2(R)

== system MATE_SynchronousMachineV2/MATE_LineCommutatedConverter/MATE_AGGREG/MATEinterface_9nodes/Simscape ==
  Electrical Reference1 : fl_lib/Electrical/Electrical Elements/Electrical Reference
  PS-S : nesl_utility/PS-Simulink Converter  PhysicalDomain=network_engine_domain  SubClassName=ps_output  LeftPortType=input  RightPortType=output  PseudoPeriodic=off  Frequencies=[]  VectorFormat=1-D array  Unit=V  AffineConversion=off
  Voltage Sensor : fl_lib/Electrical/Electrical Sensors/Voltage Sensor
  V : PMIOPort  Side=Left
  Out : Outport  VectorParamsAs1DForOutWhenUnconnected=off
  wires:
  PS-S/1 -> Out/1  "voltage"
  connections:
  Electrical Reference1/LConn1 -- Voltage Sensor/RConn2
  V/RConn1 -- Voltage Sensor/LConn1
  PS-S/LConn1 -- Voltage Sensor/RConn1

== system MATE_SynchronousMachineV2/MATE_LineCommutatedConverter/MATE_AGGREG/MATEinterface_9nodes/Simscape1 ==
  Electrical Reference1 : fl_lib/Electrical/Electrical Elements/Electrical Reference
  PS-S : nesl_utility/PS-Simulink Converter  PhysicalDomain=network_engine_domain  SubClassName=ps_output  LeftPortType=input  RightPortType=output  PseudoPeriodic=off  Frequencies=[]  VectorFormat=1-D array  Unit=V  AffineConversion=off
  Voltage Sensor : fl_lib/Electrical/Electrical Sensors/Voltage Sensor
  V : PMIOPort  Side=Left
  Out : Outport  VectorParamsAs1DForOutWhenUnconnected=off
  wires:
  PS-S/1 -> Out/1  "voltage"
  connections:
  PS-S/LConn1 -- Voltage Sensor/RConn1
  V/RConn1 -- Voltage Sensor/LConn1
  Electrical Reference1/LConn1 -- Voltage Sensor/RConn2

== system MATE_SynchronousMachineV2/MATE_LineCommutatedConverter/MATE_AGGREG/MATEinterface_9nodes/Simscape2 ==
  Electrical Reference1 : fl_lib/Electrical/Electrical Elements/Electrical Reference
  PS-S : nesl_utility/PS-Simulink Converter  PhysicalDomain=network_engine_domain  SubClassName=ps_output  LeftPortType=input  RightPortType=output  PseudoPeriodic=off  Frequencies=[]  VectorFormat=1-D array  Unit=V  AffineConversion=off
  Voltage Sensor : fl_lib/Electrical/Electrical Sensors/Voltage Sensor
  V : PMIOPort  Side=Left
  Out : Outport  VectorParamsAs1DForOutWhenUnconnected=off
  wires:
  PS-S/1 -> Out/1  "voltage"
  connections:
  Electrical Reference1/LConn1 -- Voltage Sensor/RConn2
  V/RConn1 -- Voltage Sensor/LConn1
  PS-S/LConn1 -- Voltage Sensor/RConn1

== system MATE_SynchronousMachineV2/MATE_LineCommutatedConverter/MATE_AGGREG/MATEinterface_9nodes/Simscape3 ==
  Electrical Reference1 : fl_lib/Electrical/Electrical Elements/Electrical Reference
  PS-S : nesl_utility/PS-Simulink Converter  PhysicalDomain=network_engine_domain  SubClassName=ps_output  LeftPortType=input  RightPortType=output  PseudoPeriodic=off  Frequencies=[]  VectorFormat=1-D array  Unit=V  AffineConversion=off
  Voltage Sensor : fl_lib/Electrical/Electrical Sensors/Voltage Sensor
  V : PMIOPort  Side=Left
  Out : Outport  VectorParamsAs1DForOutWhenUnconnected=off
  wires:
  PS-S/1 -> Out/1  "voltage"
  connections:
  PS-S/LConn1 -- Voltage Sensor/RConn1
  V/RConn1 -- Voltage Sensor/LConn1
  Electrical Reference1/LConn1 -- Voltage Sensor/RConn2

== system MATE_SynchronousMachineV2/MATE_LineCommutatedConverter/MATE_AGGREG/MATEinterface_9nodes/Simscape4 ==
  Electrical Reference1 : fl_lib/Electrical/Electrical Elements/Electrical Reference
  PS-S : nesl_utility/PS-Simulink Converter  PhysicalDomain=network_engine_domain  SubClassName=ps_output  LeftPortType=input  RightPortType=output  PseudoPeriodic=off  Frequencies=[]  VectorFormat=1-D array  Unit=V  AffineConversion=off
  Voltage Sensor : fl_lib/Electrical/Electrical Sensors/Voltage Sensor
  V : PMIOPort  Side=Left
  Out : Outport  VectorParamsAs1DForOutWhenUnconnected=off
  wires:
  PS-S/1 -> Out/1  "voltage"
  connections:
  Electrical Reference1/LConn1 -- Voltage Sensor/RConn2
  V/RConn1 -- Voltage Sensor/LConn1
  PS-S/LConn1 -- Voltage Sensor/RConn1

== system MATE_SynchronousMachineV2/MATE_LineCommutatedConverter/MATE_AGGREG/MATEinterface_9nodes/Voltage Source ==
  I : Inport
  Controlled Current Source1 : fl_lib/Electrical/Electrical Sources/Controlled Current Source
  Simulink-PS Converter : nesl_utility/Simulink-PS Converter  PhysicalDomain=network_engine_domain  SubClassName=ps_input  LeftPortType=input  RightPortType=output  PseudoPeriodic=off  Frequencies=[]  NoiseDistribution=none  NoiseParameters=[]  Unit=1  AffineConversion=off  FilteringAndDerivatives=zero  SimscapeFilterOrder=1  InputFilterTimeConstant=.001  UdotUserProvided=0
  + : PMIOPort  Side=Right
  - : PMIOPort  Port=2  Side=Right
  wires:
  I/1 -> Simulink-PS Converter/1
  connections:
  Controlled Current Source1/LConn1 -- +/RConn1
  Controlled Current Source1/RConn2 -- -/RConn1
  Controlled Current Source1/RConn1 -- Simulink-PS Converter/RConn1

== system MATE_SynchronousMachineV2/MATE_LineCommutatedConverter/MATE_AGGREG/MATEinterface_9nodes/Voltage Source1 ==
  I : Inport
  Controlled Current Source1 : fl_lib/Electrical/Electrical Sources/Controlled Current Source
  Simulink-PS Converter : nesl_utility/Simulink-PS Converter  PhysicalDomain=network_engine_domain  SubClassName=ps_input  LeftPortType=input  RightPortType=output  PseudoPeriodic=off  Frequencies=[]  NoiseDistribution=none  NoiseParameters=[]  Unit=1  AffineConversion=off  FilteringAndDerivatives=zero  SimscapeFilterOrder=1  InputFilterTimeConstant=.001  UdotUserProvided=0
  + : PMIOPort  Side=Right
  - : PMIOPort  Port=2  Side=Right
  wires:
  I/1 -> Simulink-PS Converter/1
  connections:
  Controlled Current Source1/RConn1 -- Simulink-PS Converter/RConn1
  Controlled Current Source1/RConn2 -- -/RConn1
  Controlled Current Source1/LConn1 -- +/RConn1

== system MATE_SynchronousMachineV2/MATE_LineCommutatedConverter/MATE_AGGREG/MATEinterface_9nodes/Voltage Source2 ==
  I : Inport
  Controlled Current Source1 : fl_lib/Electrical/Electrical Sources/Controlled Current Source
  Simulink-PS Converter : nesl_utility/Simulink-PS Converter  PhysicalDomain=network_engine_domain  SubClassName=ps_input  LeftPortType=input  RightPortType=output  PseudoPeriodic=off  Frequencies=[]  NoiseDistribution=none  NoiseParameters=[]  Unit=1  AffineConversion=off  FilteringAndDerivatives=zero  SimscapeFilterOrder=1  InputFilterTimeConstant=.001  UdotUserProvided=0
  + : PMIOPort  Side=Right
  - : PMIOPort  Port=2  Side=Right
  wires:
  I/1 -> Simulink-PS Converter/1
  connections:
  Controlled Current Source1/LConn1 -- +/RConn1
  Controlled Current Source1/RConn2 -- -/RConn1
  Controlled Current Source1/RConn1 -- Simulink-PS Converter/RConn1

== system MATE_SynchronousMachineV2/MATE_LineCommutatedConverter/MATE_AGGREG/MATEinterface_9nodes/Voltage Source3 ==
  I : Inport
  Controlled Current Source1 : fl_lib/Electrical/Electrical Sources/Controlled Current Source
  Simulink-PS Converter : nesl_utility/Simulink-PS Converter  PhysicalDomain=network_engine_domain  SubClassName=ps_input  LeftPortType=input  RightPortType=output  PseudoPeriodic=off  Frequencies=[]  NoiseDistribution=none  NoiseParameters=[]  Unit=1  AffineConversion=off  FilteringAndDerivatives=zero  SimscapeFilterOrder=1  InputFilterTimeConstant=.001  UdotUserProvided=0
  + : PMIOPort  Side=Right
  - : PMIOPort  Port=2  Side=Right
  wires:
  I/1 -> Simulink-PS Converter/1
  connections:
  Controlled Current Source1/RConn1 -- Simulink-PS Converter/RConn1
  Controlled Current Source1/RConn2 -- -/RConn1
  Controlled Current Source1/LConn1 -- +/RConn1

== system MATE_SynchronousMachineV2/MATE_LineCommutatedConverter/MATE_AGGREG/MATEinterface_9nodes/Voltage Source4 ==
  I : Inport
  Controlled Current Source1 : fl_lib/Electrical/Electrical Sources/Controlled Current Source
  Simulink-PS Converter : nesl_utility/Simulink-PS Converter  PhysicalDomain=network_engine_domain  SubClassName=ps_input  LeftPortType=input  RightPortType=output  PseudoPeriodic=off  Frequencies=[]  NoiseDistribution=none  NoiseParameters=[]  Unit=1  AffineConversion=off  FilteringAndDerivatives=zero  SimscapeFilterOrder=1  InputFilterTimeConstant=.001  UdotUserProvided=0
  + : PMIOPort  Side=Right
  - : PMIOPort  Port=2  Side=Right
  wires:
  I/1 -> Simulink-PS Converter/1
  connections:
  Controlled Current Source1/LConn1 -- +/RConn1
  Controlled Current Source1/RConn2 -- -/RConn1
  Controlled Current Source1/RConn1 -- Simulink-PS Converter/RConn1

== system MATE_SynchronousMachineV2/turbine1/Hydraulic Turbine and Governor/Model/Discrete PID Controller ==
  note: Discrete PID Controller
  note: Pierre Giroux, Gilbert Sybille
      | Power System Simulation Laboratory
      | IREQ, Hydro-Quebc
  Error : Inport
  "Derivative " : DiscreteTransferFcn  Numerator=[2 -2]  Denominator=[Ts+2*TcD Ts-2*TcD]  SampleTime=Ts
  Discrete-Time Integrator : DiscreteIntegrator  InitialCondition=Init  SampleTime=Ts  LimitOutput=on  UpperSaturationLimit=UpperLimit  LowerSaturationLimit=LowerLimit  ICPrevOutput=DiscIntNeverNeededParam  ICPrevScaledInput=DiscIntNeverNeededParam
  Kp4 : Gain  Gain=Kp  SaturateOnIntegerOverflow=on  OutDataTypeStr=Inherit: Same as input  ParamDataTypeStr=Inherit: Same as input
  Kp5 : Gain  Gain=Ki  SaturateOnIntegerOverflow=on  OutDataTypeStr=Inherit: Same as input  ParamDataTypeStr=Inherit: Same as input
  Kp6 : Gain  Gain=Kd  SaturateOnIntegerOverflow=on  OutDataTypeStr=Inherit: Same as input  ParamDataTypeStr=Inherit: Same as input
  Saturation2 : Saturate  UpperLimit=UpperLimit  LowerLimit=LowerLimit
  Sum6 : Sum  Inputs=+++  InputSameDT=on  SaturateOnIntegerOverflow=on  OutDataTypeStr=Inherit: Same as first input
  Out : Outport  InitialOutput=0
  wires:
  Error/1 -> Kp4/1, Kp5/1, Kp6/1
  Sum6/1 -> Saturation2/1
  Kp5/1 -> Discrete-Time Integrator/1
  Kp6/1 -> "Derivative "/1
  Kp4/1 -> Sum6/1
  Discrete-Time Integrator/1 -> Sum6/2
  "Derivative "/1 -> Sum6/3
  Saturation2/1 -> Out/1

== system MATE_SynchronousMachineV2/turbine1/Hydraulic Turbine and Governor/Model/servo-motor ==
  regulator's output : Inport
  Sum4 : Sum  Inputs=+-  InputSameDT=on  SaturateOnIntegerOverflow=on  OutDataTypeStr=Inherit: Same as first input
  position : DiscreteIntegrator  InitialCondition=go  SampleTime=Ts  LimitOutput=on  UpperSaturationLimit=gmax  LowerSaturationLimit=gmin  ICPrevOutput=DiscIntNeverNeededParam  ICPrevScaledInput=DiscIntNeverNeededParam
  servo-motor : Subsystem
  speed limit : Saturate  UpperLimit=vgmax  LowerLimit=vgmin
  gate opening : Outport  InitialOutput=0
  wires:
  position/1 -> Sum4/2, gate opening/1
  speed limit/1 -> position/1
  servo-motor/1(Out) -> speed limit/1
  Sum4/1 -> servo-motor/1(In)
  regulator's output/1 -> Sum4/1

== system MATE_SynchronousMachineV2/turbine1/Hydraulic Turbine and Governor/Model/turbine ==
  dw : Inport
  gate opening : Inport  Port=2
  Constant : Constant
  Fcn : Fcn  Expr=(u(2)/u(1))^2
  Gain2 : Gain  Gain=1/tw  SaturateOnIntegerOverflow=on  OutDataTypeStr=Inherit: Same as input  ParamDataTypeStr=Inherit: Same as input
  Mux : Mux  Inputs=2
  Product : Product  InputSameDT=on  SaturateOnIntegerOverflow=on  OutDataTypeStr=Inherit: Same as first input
  Sum2 : Sum  Inputs=-+  InputSameDT=on  SaturateOnIntegerOverflow=on  OutDataTypeStr=Inherit: Same as first input
  Sum3 : Sum  Inputs=-+  InputSameDT=on  SaturateOnIntegerOverflow=on  OutDataTypeStr=Inherit: Same as first input
  beta : Gain  Gain=beta  SaturateOnIntegerOverflow=on  OutDataTypeStr=Inherit: Same as input  ParamDataTypeStr=Inherit: Same as input
  position : DiscreteIntegrator  InitialCondition=po  SampleTime=Ts  UpperSaturationLimit=0  LowerSaturationLimit=0  ICPrevOutput=DiscIntNeverNeededParam  ICPrevScaledInput=DiscIntNeverNeededParam
  turbine gain : Gain  Gain=1/(gmax-gmin)  SaturateOnIntegerOverflow=on  OutDataTypeStr=Inherit: Same as input  ParamDataTypeStr=Inherit: Same as input
  Pm : Outport  InitialOutput=0
  wires:
  turbine gain/1 -> Mux/1
  gate opening/1 -> turbine gain/1
  Mux/1 -> Fcn/1
  Fcn/1 -> Sum2/2
  Constant/1 -> Sum3/2
  Product/1 -> Pm/1
  Sum3/1 -> Gain2/1
  Gain2/1 -> position/1
  Sum2/1 -> Sum3/1, Product/1
  beta/1 -> Sum2/1
  dw/1 -> beta/1
  position/1 -> Product/2, Mux/2

== system MATE_SynchronousMachineV2/Command/Synchro Generateur d'mpulsions /Discrete 3-phase PLL/Automatic Gain Control/3-phase PLL-Driven Positive-Sequence Fundamental Value ==
  note: Discrete 3-phase PLL-Driven Positive-Sequence Fundamental Value
  note: Pierre Giroux, Gilbert Sybille
      | Power System Simulation Laboratory
      | IREQ, Hydro-Quebc
  Freq : Inport
  Sin_Cos : Inport  Port=2  PortDimensions=2
  abc : Inport  Port=3  PortDimensions=3
  Cartesian to Polar : simulink_extras/Transformations/Cartesian to Polar
  Demux : Demux  Outputs=3
      settings: DisplayOption=none
  Discrete Variable Frequency Mean value : Subsystem  mask(Discrete Variable-Frequency Mean Value){Finit=Finit, Fmin=Fmin, Vinit=Real_Init, Ts=Ts}
      mask prompts: Finit "Initial frequency (Hz):"; Fmin "Minimum frequency (Hz):"; Vinit "Initial input (DC component):"; Ts "Sample time:"
      mask help: Compute the mean value of input 2 over a running window of one cycle of frequency given by input 1.
      mask init:
      | MaxDelay=1/Fmin+Ts;
      mask Display: disp('')
  Discrete Variable Frequency Mean value2 : Subsystem  mask(Discrete Variable-Frequency Mean Value){Finit=Finit, Fmin=Fmin, Vinit=Imag_Init, Ts=Ts}
      mask prompts: Finit "Initial frequency (Hz):"; Fmin "Minimum frequency (Hz):"; Vinit "Initial input (DC component):"; Ts "Sample time:"
      mask help: Compute the mean value of input 2 over a running window of one cycle of frequency given by input 1.
      mask init:
      | MaxDelay=1/Fmin+Ts;
      mask Display: disp('')
  Rad->Deg. : Gain  Gain=180/pi  SaturateOnIntegerOverflow=on  OutDataTypeStr=Inherit: Same as input  ParamDataTypeStr=Inherit: Same as input
  Terminator : Terminator
  abc_to_dq0 Transformation : Subsystem  mask(abc to dq0 Transformation){}
      mask help: Perform a Park transformation from the three-phase (abc) reference frame to the dq0 reference frame.
      mask Display: disp('')
  Mag : Outport  VectorParamsAs1DForOutWhenUnconnected=off
  Phase : Outport  Port=2  VectorParamsAs1DForOutWhenUnconnected=off
  wires:
  Cartesian to Polar/2 -> Rad->Deg./1
  Cartesian to Polar/1 -> Mag/1
  Demux/3 -> Terminator/1
  abc_to_dq0 Transformation/1(dq0) -> Demux/1
  abc/1 -> abc_to_dq0 Transformation/1(abc)
  Demux/1 -> Discrete Variable Frequency Mean value/2(In)
  Demux/2 -> Discrete Variable Frequency Mean value2/2(In)
  Discrete Variable Frequency Mean value2/1(Mean) -> Cartesian to Polar/2  "Real"
  Rad->Deg./1 -> Phase/1
  Discrete Variable Frequency Mean value/1(Mean) -> Cartesian to Polar/1  "Real"
  Freq/1 -> Discrete Variable Frequency Mean value2/1(Freq), Discrete Variable Frequency Mean value/1(Freq)
  Sin_Cos/1 -> abc_to_dq0 Transformation/2(sin_cos)

== system MATE_SynchronousMachineV2/Command/Synchro Generateur d'mpulsions /Discrete 3-phase PLL/Variable Frequency Mean value/Correction subsystem ==
  N : Inport
  F : Inport  Port=2
  In : Inport  Port=3
  Gain1 : Gain  Gain=0.5  SaturateOnIntegerOverflow=on  OutDataTypeStr=Inherit: Same as input  ParamDataTypeStr=Inherit: Same as input
  Product2 : Product  Inputs=*/  InputSameDT=on  SaturateOnIntegerOverflow=on  OutDataTypeStr=Inherit: Same as first input
  Product4 : Product  Inputs=**  InputSameDT=on  SaturateOnIntegerOverflow=on  OutDataTypeStr=Inherit: Same as first input
  Product5 : Product  Inputs=**  InputSameDT=on  SaturateOnIntegerOverflow=on  OutDataTypeStr=Inherit: Same as first input
  Sum1 : Sum  Inputs=+-  InputSameDT=on  SaturateOnIntegerOverflow=on  OutDataTypeStr=Inherit: Same as first input
  Sum4 : Sum  InputSameDT=on  SaturateOnIntegerOverflow=on  OutDataTypeStr=Inherit: Same as first input
  Sum5 : Sum  Inputs=+-  InputSameDT=on  SaturateOnIntegerOverflow=on  OutDataTypeStr=Inherit: Same as first input
  Unit Delay : UnitDelay  SampleTime=Ts  HasFrameUpgradeWarning=on
  Out : Outport  VectorParamsAs1DForOutWhenUnconnected=off
  wires:
  Unit Delay/1 -> Sum1/2
  N/1 -> Sum5/1, Product2/2
  F/1 -> Sum5/2
  Sum5/1 -> Product2/1, Product5/1
  Product2/1 -> Product4/1
  In/1 -> Sum1/1, Unit Delay/1, Sum4/2
  Sum1/1 -> Product5/2
  Product5/1 -> Gain1/1
  Gain1/1 -> Sum4/1
  Sum4/1 -> Product4/2
  Product4/1 -> Out/1

== system MATE_SynchronousMachineV2/Command/Synchro Generateur d'mpulsions /Discrete 3-phase PLL/Variable Frequency Mean value/Discrete Variable Transport Delay ==
  In : Inport
  D : Inport  Port=2
  "S-Function " : S-Function  FunctionName=discreteVariableTransportDelay  Parameters=MaxDelay,Ts,InitialValue  SFunctionDeploymentMode=off  EnableBusSupport=off
  Out : Outport  VectorParamsAs1DForOutWhenUnconnected=off
  wires:
  "S-Function "/1 -> Out/1
  In/1 -> "S-Function "/1
  D/1 -> "S-Function "/2

== system MATE_SynchronousMachineV2/Command/Synchro Generateur d'mpulsions /Discrete Synchronized 12-Pulse Generator/Pulse generation/12 Flip-Flops ==
  S : Inport
  R : Inport  Port=2
  6 Flip-Flop : Subsystem
  6 Flip-Flop1 : Subsystem
  Demux : Demux  Outputs=2
      settings: DisplayOption=none
  Demux1 : Demux  Outputs=2
      settings: DisplayOption=none
  Mux : Mux  Inputs=2
  Q : Outport  VectorParamsAs1DForOutWhenUnconnected=off
  wires:
  S/1 -> Demux/1
  Demux/1 -> 6 Flip-Flop/1(S)
  Demux/2 -> 6 Flip-Flop1/1(S)
  R/1 -> Demux1/1
  Demux1/2 -> 6 Flip-Flop1/2(R)
  Demux1/1 -> 6 Flip-Flop/2(R)
  6 Flip-Flop/1(Q) -> Mux/1
  Mux/1 -> Q/1
  6 Flip-Flop1/1(Q) -> Mux/2
